simulink model "Q2sim"  (R2019b)
settings: Solver=VariableStepAuto  StartTime=0.0  StopTime=511  RelTol=1e-3
model workspace (MATLAB code in the model file):
  | %%
  | %Generating the input signal
  | Bmax=0.2;
  | Range=[-1,1];
  | N=2555;
  | Ts=0.2;
  | u1=idinput(N,'prbs',[0,Bmax],Range);
  | uin = [(0:1:length(u1)-1)'*Ts (u1)];
settings Model: OrderedModelArguments=off  Creator=Raj  LastModifiedBy=Raj

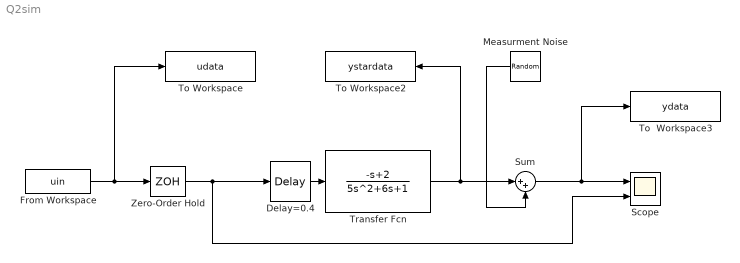
== system Q2sim ==
  Delay=0.4 : TransportDelay  DelayTime=0.4
  "From Workspace " : FromWorkspace  VariableName=uin  SampleTime=0.2
  Measurment Noise : RandomNumber  Variance=0.1  SampleTime=0.1
  "Scope " : Scope  NumInputPorts=2
  Sum : Sum  Inputs=|++
  To  Workspace3 : ToWorkspace  VariableName=ydata  SaveFormat=Timeseries  SampleTime=0.2
  "To Workspace " : ToWorkspace  VariableName=udata  SaveFormat=Timeseries  SampleTime=0.2
  "To Workspace2  " : ToWorkspace  VariableName=ystardata  SaveFormat=Timeseries  SampleTime=0.2
  "Transfer Fcn " : TransferFcn  Numerator=[-1 2]  Denominator=[5 6 1]
  "Zero-Order Hold " : ZeroOrderHold  SampleTime=-1
  wires:
  Delay=0.4/1 -> "Transfer Fcn "/1
  "Zero-Order Hold "/1 -> "Scope "/2, Delay=0.4/1
  "From Workspace "/1 -> "To Workspace "/1, "Zero-Order Hold "/1
  "Transfer Fcn "/1 -> "To Workspace2  "/1, Sum/1
  Measurment Noise/1 -> Sum/2
  Sum/1 -> To  Workspace3/1, "Scope "/1
